simulink model "water_4hopper_open"  (Simulink 8.0)
settings: Solver=ode23  StartTime=0.0  StopTime=30  RelTol=1e-4
values from neighbouring files (symbols this model uses):
  alpha = 30    [SimParam_4VDF.m]
  C_d = 0.703    [SimParam_4VDF.m]
  density = 1000    [SimParam_4VDF.m]
  dTorqueAmp = 0    [SimParam_4VDF.m]
  dTorqueFreq = 0.5    [SimParam_4VDF.m]
  dTorquePhase = 2*pi*rand(1,4)    [SimParam_4VDF.m]
  frame_inertia = diag([Ix,Iy,Iz])    [SimParam_4VDF.m]
  freq = 60    [SimParam_4VDF.m]
  g = 9.81    [SimParam_4VDF.m]
  leg_length = 0.0249    [SimParam_4VDF.m]
  mass = 0.1    [SimParam_4VDF.m]
  S1 = pi*r1^2*0.9185    (= 0.00115422114093)    [SimParam_4VDF.m]
  S2 = pi*r2^2*0.9185    (= 7.21388213081e-05)    [SimParam_4VDF.m]
  tau = 0.005    [SimParam_4VDF.m]
  waveAmp = 0    [SimParam_4VDF.m]
  waveFreq = 0.5    [SimParam_4VDF.m]
undefined symbols (not defined in the file): amp, cw_FL_HL, cw_FR_FL, cw_FR_HR, cw_HR_HL, FL_HL_lag, FR_FL_lag, FR_HR_lag, HR_HL_lag, wavePhase, y_0
libraries: mblibv1 x33
(part 2 of 2)

== system water_4hopper_open/CPG_Network2/split FL3/enable ==
  in : Inport
  Constant1 : Constant
  Constant2 : Constant
  Derivative : Derivative
  Gain : Gain  Gain=.5
  Gain1 : Gain  Gain=.5
  Sign : Signum
  Sum1 : Sum  Inputs=|++
  Sum2 : Sum  Inputs=|-+
  pos : Outport
  neg : Outport  Port=2
  wires:
  Derivative/1 -> Sign/1
  Constant1/1 -> Sum1/2
  Sign/1 -> Sum2/1, Sum1/1
  Gain/1 -> pos/1
  in/1 -> Derivative/1
  Sum1/1 -> Gain/1
  Constant2/1 -> Sum2/2
  Gain1/1 -> neg/1
  Sum2/1 -> Gain1/1
